simulink model "d1"  (R2013a)
settings: Solver=ode45  StartTime=0.0  StopTime=100.0  FixedStep=0.01  MaxStep=0.001  RelTol=1e-3
undefined symbols (not defined in the file): k1, Tp1
settings Model: Creator=adasdeb  LastModifiedBy=adasdeb
settings DataIOCC: LimitDataPoints=off

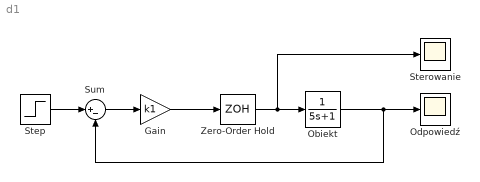
== system d1 ==
  Gain : Gain  Gain=k1
  Obiekt : TransferFcn  Denominator=[5 1]
  Odpowiedź : Scope
      settings: SaveName=resp1
  Step : Step  SampleTime=0
  Sterowanie : Scope
      settings: SaveName=ster1
  Sum : Sum  Inputs=|+-
  Zero-Order Hold : ZeroOrderHold  SampleTime=Tp1
  wires:
  Sum/1 -> Gain/1
  Gain/1 -> Zero-Order Hold/1
  Zero-Order Hold/1 -> Sterowanie/1, Obiekt/1
  Step/1 -> Sum/1
  Obiekt/1 -> Odpowiedź/1, Sum/2
